simulink model "SLFLPUCSI"  (R2016a)
settings: Solver=VariableStepAuto  StartTime=0.0  StopTime=4/50  MaxStep=1e-6  MinStep=1e-7  RelTol=1e-3
libraries: powerlib x11, simulink x4
settings Model: Creator=satheeshwaran  LastModifiedBy=satheeshwaran

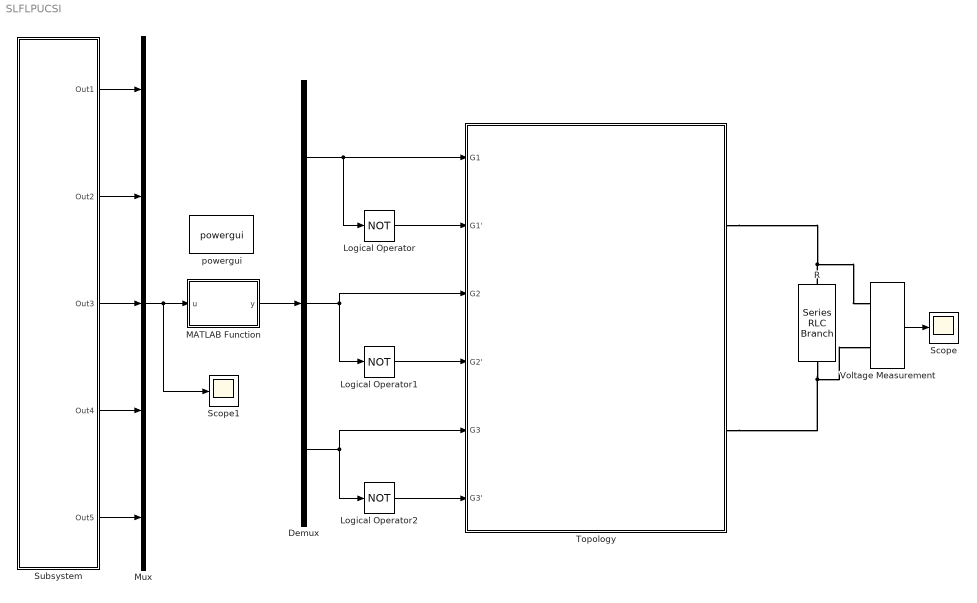
== system SLFLPUCSI ==
  Demux : Demux  Outputs=3
  Logical Operator : Logic  Operator=NOT  AllPortsSameDT=off  OutDataTypeStr=boolean
  Logical Operator1 : Logic  Operator=NOT  AllPortsSameDT=off  OutDataTypeStr=boolean
  Logical Operator2 : Logic  Operator=NOT  AllPortsSameDT=off  OutDataTypeStr=boolean
  MATLAB Function : MATLAB Function  TreatAsAtomicUnit=on
  Mux : Mux  Inputs=5
  R : powerlib/Elements/Series RLC Branch  LConnTagsString=__new0  RConnTagsString=__new0  BranchType=R  Resistance=100  Inductance=1e-3  SetiL0=off  InitialCurrent=0  Capacitance=1e-6  Setx0=off  InitialVoltage=0  Measurements=None
  Scope : Scope
  Scope1 : Scope
  Subsystem : Subsystem
  Topology : Subsystem
  Voltage Measurement : powerlib/Measurements/Voltage Measurement  PhasorSimulation=off  OutputType=Complex  PSBequivalent=0
  powergui : powerlib/powergui  Priority=1  SimulationMode=Continuous  SolverType=Tustin/Backward Euler (TBE)  SampleTime=50e-6  frequency=60  SPID=off  DisableSnubberDevices=off  DisableRonSwitches=off  DisableVfSwitches=off  SwTol=0  DisplayEquations=off  Interpol=off  ExternalGateDelay=off  methode=off  Ts=10  FunctionMessages=off  echomessages=off  HookPort=off  EnableUseOfTLC=off  x0status=blocks  frequencyindice=0  Pbase=100e6  ErrMax=1e-4  Iterations=50  UnitsV=kV  UnitsW=MW  buscounter=0  RestoreLinks=warning  ResistiveCurrentMeasurement=off  Frange=[0:2:500]  Ylog=off  Xlog=on  ShowGrid=off  save=off  variable=ZData  structure=load  ZoomFFT=off  StartTime=0.04  cycles=1  DisplayStyle=1  fundamental=50  FreqAxis=off  MaxFrequency=10000  frequencyindicesteady=1  RmsSteady=1  display=off
  wires:
  Voltage Measurement/1 -> Scope/1
  MATLAB Function/1(y) -> Demux/1
  Mux/1 -> Scope1/1, MATLAB Function/1(u)
  Demux/1 -> Logical Operator/1, Topology/1(G1)
  Demux/3 -> Topology/5(G3), Logical Operator2/1
  Demux/2 -> Logical Operator1/1, Topology/3(G2)
  Subsystem/1(Out1) -> Mux/1
  Subsystem/2(Out2) -> Mux/2
  Subsystem/3(Out3) -> Mux/3
  Subsystem/4(Out4) -> Mux/4
  Subsystem/5(Out5) -> Mux/5
  Logical Operator/1 -> Topology/2(G1')
  Logical Operator1/1 -> Topology/4(G2')
  Logical Operator2/1 -> Topology/6(G3')
  connections:
  R/LConn1 -- Topology/RConn1 -- Voltage Measurement/LConn1
  Topology/RConn2 -- R/RConn1 -- Voltage Measurement/LConn2

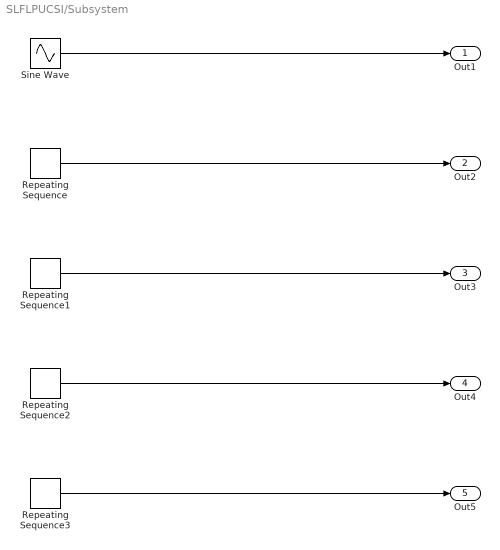
== system SLFLPUCSI/Subsystem ==
  Repeating Sequence : simulink/Sources/Repeating Sequence  rep_seq_t=[0 1/4000 1/2000]  rep_seq_y=[0.5 1 0.5]
  Repeating Sequence1 : simulink/Sources/Repeating Sequence  rep_seq_t=[0 1/4000 1/2000]  rep_seq_y=[0 0.5 0]
  Repeating Sequence2 : simulink/Sources/Repeating Sequence  rep_seq_t=[0 1/4000 1/2000]  rep_seq_y=[-0.5 0 -0.5]
  Repeating Sequence3 : simulink/Sources/Repeating Sequence  rep_seq_t=[0 1/4000 1/2000]  rep_seq_y=[-1 -0.5 -1]
  Sine Wave : Sin  Frequency=2*pi*50  SampleTime=0
  Out1 : Outport
  Out2 : Outport  Port=2
  Out3 : Outport  Port=3
  Out4 : Outport  Port=4
  Out5 : Outport  Port=5
  wires:
  Sine Wave/1 -> Out1/1
  Repeating Sequence/1 -> Out2/1
  Repeating Sequence1/1 -> Out3/1
  Repeating Sequence3/1 -> Out5/1
  Repeating Sequence2/1 -> Out4/1

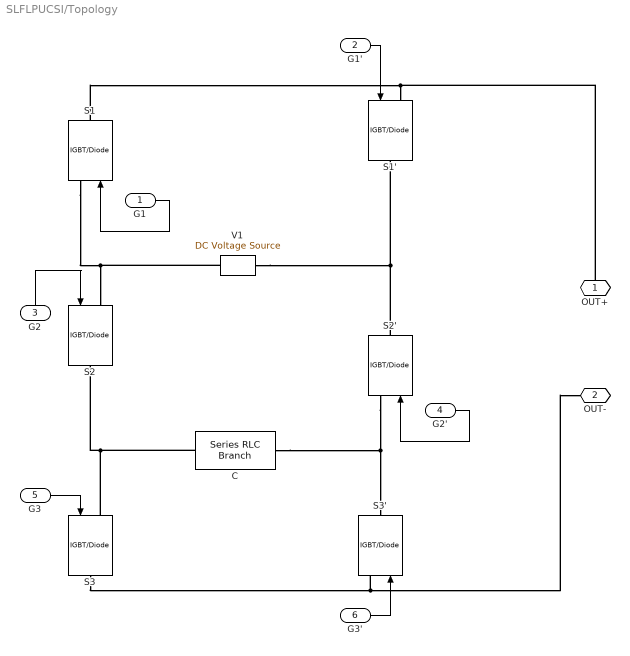
== system SLFLPUCSI/Topology ==
  G1 : Inport
  G1' : Inport  Port=2
  G2 : Inport  Port=3
  G2' : Inport  Port=4
  G3 : Inport  Port=5
  G3' : Inport  Port=6
  C : powerlib/Elements/Series RLC Branch  LConnTagsString=__new0  RConnTagsString=__new0  BranchType=C  Resistance=1  Inductance=1e-3  SetiL0=off  InitialCurrent=0  Capacitance=0.0025  Setx0=off  InitialVoltage=0  Measurements=None
  S1 : powerlib/Power Electronics/IGBT//Diode  Ron=1e-3  Rs=1e5  Cs=inf  Measurements=off
  S1' : powerlib/Power Electronics/IGBT//Diode  Ron=1e-3  Rs=1e5  Cs=inf  Measurements=off
  S2 : powerlib/Power Electronics/IGBT//Diode  Ron=1e-3  Rs=1e5  Cs=inf  Measurements=off
  S2' : powerlib/Power Electronics/IGBT//Diode  Ron=1e-3  Rs=1e5  Cs=inf  Measurements=off
  S3 : powerlib/Power Electronics/IGBT//Diode  Ron=1e-3  Rs=1e5  Cs=inf  Measurements=off
  S3' : powerlib/Power Electronics/IGBT//Diode  Ron=1e-3  Rs=1e5  Cs=inf  Measurements=off
  V1 : powerlib/Electrical Sources/DC Voltage Source  Amplitude=200  Measurements=None
  OUT+ : PMIOPort  Port=1  Side=Right
  OUT- : PMIOPort  Port=2  Side=Right
  wires:
  G2/1 -> S2/1
  G3/1 -> S3/1
  G1/1 -> S1/1
  G2'/1 -> S2'/1
  G3'/1 -> S3'/1
  G1'/1 -> S1'/1
  connections:
  S2'/LConn1 -- S3'/RConn1 -- C/RConn1
  S1/RConn1 -- OUT+/RConn1 -- S1'/LConn1
  V1/LConn1 -- S2'/RConn1 -- S1'/RConn1
  S3/RConn1 -- OUT-/RConn1 -- S3'/LConn1
  C/LConn1 -- S3/LConn1 -- S2/RConn1
  V1/RConn1 -- S1/LConn1 -- S2/LConn1

== matlab function SLFLPUCSI/MATLAB Function ==
  data: u input; y output
function y = fcn(u)
sine = u(1);
c1 = u(2);
c2 = u(3);
c3 = u(4);
c4 = u(5);

s1 = 0;
s2 = 0;
s3 = 0;

if(sine >= c1)
    s1=1;
end
if(sine < c1 && sine >= c2)
    s1=1;s3=1; 
end
if(sine >= 0 && (sine < c2 && sine >= c3))
    s1=1;s2=1;s3=1;
end
if(sine < 0 && (sine < c2 && sine >= c3))
    s1=0;s2=0;s3=0;
end
if(sine < c3 && sine >= c4)
    s3=1;
end
if(sine < c4)
    s2=1;s3=1;
end

y = [s1;s2;s3];
